simulink model "TDC_SMC_PD_S10x2810x29"  (R2025b)
settings: Solver=ode1be  StartTime=0.0  StopTime=1  FixedStep=0.001  MaxStep=0.01  RelTol=1e-3  EnableMultiTasking=on
values from neighbouring files (symbols this model uses):
  kd = 1.0245    [PD_final.m]
  kp = 16    [PD_final.m]
libraries: fod x3
settings Model: Creator=OMEN  LastModifiedBy=Wassim DJ
settings SolverCC: ZeroCrossControl=DisableAll  AlgebraicLoopSolver=TrustRegion
settings DataIOCC: ReturnWorkspaceOutputs=off
settings OptimizationCC: LifeSpan=inf
settings DebuggingCC: UnconnectedInputMsg=warning  UnconnectedOutputMsg=warning  UnconnectedLineMsg=warning  SFUnexpectedBacktrackingDiag=warning  SFNoUnconditionalDefaultTransitionDiag=warning  ArithmeticOperatorsInVariantConditions=warning
settings ModelReferenceCC: EnableRefExpFcnMdlSchedulingChecks=on
settings SFSimCC: SimUseLocalCustomCode=off  CustomCodeUndefinedFunction=UseInterfaceOnly
settings RTWCC: RTWUseLocalCustomCode=off  GPUComputeCapability=3.5  DLArmComputeVersion=19.05
settings CodeAppCC: StateflowObjectComments=on
settings GRTTargetCC: TargetLangStandard=C89/C90 (ANSI)
settings ConfigComp: CovMetricSettings=dw  CovSaveCumulativeToWorkspaceVar=on  CovSaveSingleToWorkspaceVar=on  CovExternalEMLEnable=off

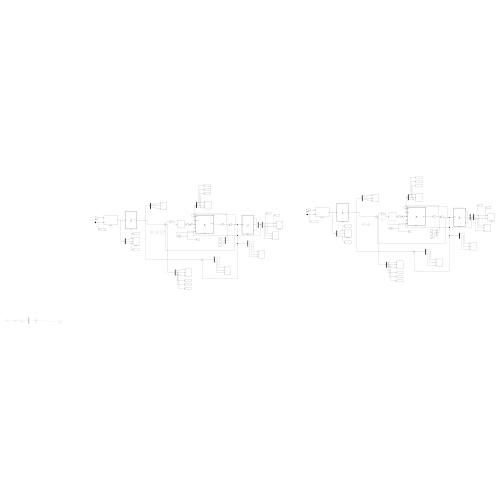
[thumbnail: Simulink's stored preview of the top-level diagram]
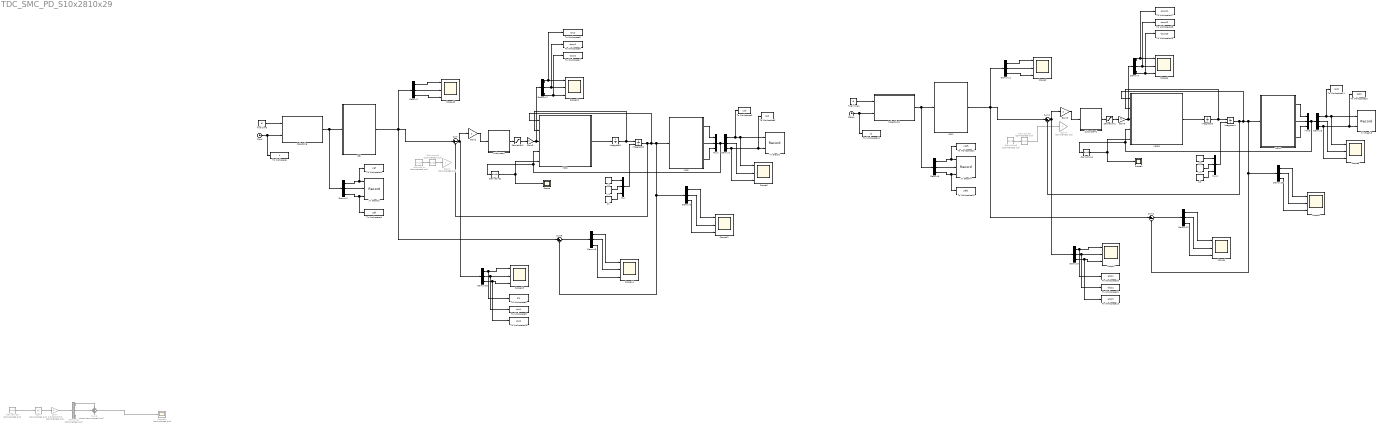
== system TDC_SMC_PD_S10x2810x29 ==
  Abs4 : Abs  Commented=on  SaturateOnIntegerOverflow=off
  Clock : Clock
  Clock1 : Clock
  Demux{1..12,17..18} (14 alike) : Demux  Outputs=3
  Demux22 : Demux  Commented=on  Outputs=3
  Derivative{,2..3,5..6} (5 alike) : Derivative  Commented=on
  Derivative1 : Derivative
  Derivative4 : Derivative
  Gain1 : Gain  Commented=on
  Gain2 : Gain
  Gain3 : Gain  Gain=3
  Gain4 : Gain  Commented=on
  Gain5 : Gain
  Gain6 : Gain  Gain=3
  Integrator1 : Integrator
  Integrator2 : Integrator  InitialConditionSource=external
  Integrator3 : Integrator
  Integrator4 : Integrator  InitialConditionSource=external
  Lam7 : Gain  Commented=on  Gain=0.000000005
  MDD : MATLAB Function  TreatAsAtomicUnit=on
  MDD1 : MATLAB Function  TreatAsAtomicUnit=on
  MGD : MATLAB Function  TreatAsAtomicUnit=on
  MGD1 : MATLAB Function  TreatAsAtomicUnit=on
  MGI : MATLAB Function  TreatAsAtomicUnit=on
  MGI1 : MATLAB Function  TreatAsAtomicUnit=on
  Mux{,1..3} (4 alike) : Mux  Inputs=3
  Saturation1 : Saturate  UpperLimit=15/12  LowerLimit=-15/12
  Saturation2 : Saturate  UpperLimit=15/12  LowerLimit=-15/12
  Scope : Scope
      settings: ActiveDisplayYMinimum=-0.16191  ActiveDisplayYMaximum=10.52394  DataLoggingVariableName=ScopeData4
  Scope1 : Scope
      settings: ActiveDisplayYMinimum=-0.16191  ActiveDisplayYMaximum=10.52394  DataLoggingVariableName=ScopeData2
  Scope{2..8,12..14,22..23} (12 alike) : Scope  NumInputPorts=3
      Scope12 settings: ActiveDisplayYMinimum=1.36342  ActiveDisplayYMaximum=5.69666
      Scope13 settings: ActiveDisplayYMinimum=-0.05003  ActiveDisplayYMaximum=2.21857  DataLoggingVariableName=ScopeData2
      Scope14 settings: ActiveDisplayYMinimum=-0.0016  ActiveDisplayYMaximum=0.00114  DataLoggingVariableName=ScopeData3
      Scope2 settings: ActiveDisplayYMinimum=1.36342  ActiveDisplayYMaximum=5.69666  DataLoggingVariableName=ScopeData3
      Scope22 settings: ActiveDisplayYMinimum=-3.78985  ActiveDisplayYMaximum=2.54114  DataLoggingVariableName=ScopeData3
      Scope23 settings: ActiveDisplayYMinimum=-0.02631  ActiveDisplayYMaximum=0.02531  DataLoggingVariableName=ScopeData4
      Scope3 settings: ActiveDisplayYMinimum=-0.05003  ActiveDisplayYMaximum=2.21857  DataLoggingVariableName=ScopeData4
      Scope4 settings: ActiveDisplayYMinimum=-0.0016  ActiveDisplayYMaximum=0.00114  DataLoggingVariableName=ScopeData5
      Scope5 settings: ActiveDisplayYMinimum=-0.31266  ActiveDisplayYMaximum=0.31251  DataLoggingVariableName=ScopeData4
      Scope6 settings: ActiveDisplayYMinimum=-4.18354  ActiveDisplayYMaximum=3.001  DataLoggingVariableName=ScopeData6
      Scope7 settings: ActiveDisplayYMinimum=-0.02631  ActiveDisplayYMaximum=0.02109  DataLoggingVariableName=ScopeData7
      Scope8 settings: ActiveDisplayYMinimum=-0.31266  ActiveDisplayYMaximum=0.31251  DataLoggingVariableName=ScopeData8
  Scope24 : Scope  Commented=on
      settings: ActiveDisplayYMinimum=-8E-7  ActiveDisplayYMaximum=7.5E-6
  Subsystem : Subsystem
  Subsystem1 : Subsystem
  Sum{,1..2,5} (4 alike) : Sum  Inputs=|+-
  Sum6 : Sum  Commented=on  Inputs=3
  To Workspace : ToWorkspace  VariableName=t  SampleTime=-1
      settings: Save2DSignal=2-D array (concatenate along first dimension)
  To Workspace1 : ToWorkspace  VariableName=xref  SampleTime=-1
      settings: Save2DSignal=2-D array (concatenate along first dimension)
  To Workspace10 : ToWorkspace  VariableName=alp2  SampleTime=-1
      settings: Save2DSignal=2-D array (concatenate along first dimension)
  To Workspace11 : ToWorkspace  VariableName=t1  SampleTime=-1
      settings: Save2DSignal=2-D array (concatenate along first dimension)
  To Workspace12 : ToWorkspace  VariableName=xref1  SampleTime=-1
      settings: Save2DSignal=2-D array (concatenate along first dimension)
  To Workspace13 : ToWorkspace  VariableName=alp13  SampleTime=-1
      settings: Save2DSignal=2-D array (concatenate along first dimension)
  To Workspace14 : ToWorkspace  VariableName=xpd1  SampleTime=-1
      settings: Save2DSignal=2-D array (concatenate along first dimension)
  To Workspace15 : ToWorkspace  VariableName=zpd1  SampleTime=-1
      settings: Save2DSignal=2-D array (concatenate along first dimension)
  To Workspace16 : ToWorkspace  VariableName=zref1  SampleTime=-1
      settings: Save2DSignal=2-D array (concatenate along first dimension)
  To Workspace17 : ToWorkspace  VariableName=coup11  SampleTime=-1
      settings: Save2DSignal=2-D array (concatenate along first dimension)
  To Workspace18 : ToWorkspace  VariableName=coup12  SampleTime=-1
      settings: Save2DSignal=2-D array (concatenate along first dimension)
  To Workspace19 : ToWorkspace  VariableName=coup13  SampleTime=-1
      settings: Save2DSignal=2-D array (concatenate along first dimension)
  To Workspace2 : ToWorkspace  VariableName=xpd  SampleTime=-1
      settings: Save2DSignal=2-D array (concatenate along first dimension)
  To Workspace20 : ToWorkspace  VariableName=alp11  SampleTime=-1
      settings: Save2DSignal=2-D array (concatenate along first dimension)
  To Workspace21 : ToWorkspace  VariableName=alp12  SampleTime=-1
      settings: Save2DSignal=2-D array (concatenate along first dimension)
  To Workspace3 : ToWorkspace  VariableName=zpd  SampleTime=-1
      settings: Save2DSignal=2-D array (concatenate along first dimension)
  To Workspace4 : ToWorkspace  VariableName=zref  SampleTime=-1
      settings: Save2DSignal=2-D array (concatenate along first dimension)
  To Workspace5 : ToWorkspace  VariableName=coup  SampleTime=-1
      settings: Save2DSignal=2-D array (concatenate along first dimension)
  To Workspace6 : ToWorkspace  VariableName=coup1  SampleTime=-1
      settings: Save2DSignal=2-D array (concatenate along first dimension)
  To Workspace7 : ToWorkspace  VariableName=coup2  SampleTime=-1
      settings: Save2DSignal=2-D array (concatenate along first dimension)
  To Workspace8 : ToWorkspace  VariableName=alp  SampleTime=-1
      settings: Save2DSignal=2-D array (concatenate along first dimension)
  To Workspace9 : ToWorkspace  VariableName=alp1  SampleTime=-1
      settings: Save2DSignal=2-D array (concatenate along first dimension)
  XY Graph1 : Record  NumPorts=2.0  FileSettingsInternal="{\"entries\":[{\"content\":{\"excelSettings\":{\"content\":{},\"type\":\"Streamout.ExcelSettings\"},\"parquetSettings\":{\"content\":{},\"type\":\"Streamout.ParquetSettings\"}},\"type\":\"Streamout.FileSettingStorage\",\"uuid\":\"\"}],\"packageUris\":[\"http:\\/\\/schema.mathworks.com\\/mf0\\/streamout_blocks\\/R2020a\"],\"version\":\"1.0\"}"  FrameSettings=[0, 0]  Layout=[1 1]  SignalsInternal="{\"entries\":[{\"content\":{\"signals\":[{\"content\":{\"blockPath\":[],\"dimensions\":[1],\"domain\":\"\",\"lineColor\":\"#a2142f\",\"plots\":[ 1 ],\"port\":1,\"signalID\":1,\"signalName\":\"Demux1:1\"},\"type\":\"RecordBlkView.Signal\",\"uuid\":\"\"},{\"content\":{\"blockPath\":[],\"dimensions\":[1],\"domain\":\"\",\"lineColor\":\"#139fff\",\"plots\":[ 1 ],\"port\":2,\"signalID\":2,\"signalName\":\"Demux1:3\"},\"type\":\"RecordBlkView.Signal\",\"uuid\":\"\"}]},\"type\":\"RecordBlkView.InputSignals\",\"uuid\":\"\"}],\"packageUris\":[\"http:\\/\\/schema.mathworks.com\\/mf0\\/streamout_blocks\\/R2020a\"],\"version\":\"1.0\"}"  VisualizationBindings="{\"xyplotplugin\":{\"info\":[{\"series\":[{\"bindingParametersList\":[{\"parameter\":\"X-Axis\",\"signalID\":1,\"signalName\":\"Demux1:1\"},{\"parameter\":\"Y-Axis\",\"signalID\":2,\"signalName\":\"Demux1:3\"}],\"seriesID\":0}],\"subplotID\":1}]}}"  CompatibilityTag=XY  st=-1
  XY Graph2 : Record  NumPorts=3.0  FileSettingsInternal="{\"entries\":[{\"content\":{\"excelSettings\":{\"content\":{},\"type\":\"Streamout.ExcelSettings\"},\"parquetSettings\":{\"content\":{},\"type\":\"Streamout.ParquetSettings\"}},\"type\":\"Streamout.FileSettingStorage\",\"uuid\":\"\"}],\"packageUris\":[\"http:\\/\\/schema.mathworks.com\\/mf0\\/streamout_blocks\\/R2020a\"],\"version\":\"1.0\"}"  FrameSettings=[0, 0, 0]  Layout=[1 1]  SignalsInternal="{\"entries\":[{\"content\":{\"signals\":[{\"content\":{\"blockPath\":[],\"dimensions\":[1,1],\"domain\":\"\",\"lineColor\":\"#a2142f\",\"plots\":[ 1 ],\"port\":1,\"signalID\":1,\"signalName\":\"Demux2:1\"},\"type\":\"RecordBlkView.Signal\",\"uuid\":\"\"},{\"content\":{\"blockPath\":[],\"dimensions\":[1,1],\"domain\":\"\",\"lineColor\":\"#139fff\",\"plots\":[ 1 ],\"port\":2,\"signalID\":2,\"signalName\":\"Demux2:2\"},\"type\":\"RecordBlkView.Signal\",\"uuid\":\"\"},{\"content\":{\"blockPath\":[],\"dimensions\":[1,1],\"domain\":\"\",\"lineColor\":\"#139fff\",\"lineWidth\":2,\"port\":3,\"signalID\":3,\"signalName\":\"Demux2:3\"},\"type\":\"RecordBlkView.Signal\",\"uuid\":\"\"}]},\"type\":\"RecordBlkView.InputSignals\",\"uuid\":\"\"}],\"packageUris\":[\"http:\\/\\/schema.mathworks.com\\/mf0\\/streamout_blocks\\/R2020a\"],\"version\":\"1.0\"}"  VisualizationBindings="{\"xyplotplugin\":{\"info\":[{\"series\":[{\"bindingParametersList\":[{\"parameter\":\"X-Axis\",\"signalID\":1,\"signalName\":\"Demux2:1\"},{\"parameter\":\"Y-Axis\",\"signalID\":2,\"signalName\":\"Demux2:2\"}],\"seriesID\":0}],\"subplotID\":1}]}}"  CompatibilityTag=XY  st=-1
  XY Graph3 : Record  NumPorts=2.0  FileSettingsInternal="{\"entries\":[{\"content\":{\"excelSettings\":{\"content\":{},\"type\":\"Streamout.ExcelSettings\"},\"parquetSettings\":{\"content\":{},\"type\":\"Streamout.ParquetSettings\"}},\"type\":\"Streamout.FileSettingStorage\",\"uuid\":\"\"}],\"packageUris\":[\"http:\\/\\/schema.mathworks.com\\/mf0\\/streamout_blocks\\/R2020a\"],\"version\":\"1.0\"}"  FrameSettings=[0, 0]  Layout=[1 1]  SignalsInternal="{\"entries\":[{\"content\":{\"signals\":[{\"content\":{\"blockPath\":[],\"dimensions\":[1],\"domain\":\"\",\"lineColor\":\"#a2142f\",\"plots\":[ 1 ],\"port\":1,\"signalID\":1,\"signalName\":\"Demux3:1\"},\"type\":\"RecordBlkView.Signal\",\"uuid\":\"\"},{\"content\":{\"blockPath\":[],\"dimensions\":[1],\"domain\":\"\",\"lineColor\":\"#139fff\",\"plots\":[ 1 ],\"port\":2,\"signalID\":2,\"signalName\":\"Demux3:3\"},\"type\":\"RecordBlkView.Signal\",\"uuid\":\"\"}]},\"type\":\"RecordBlkView.InputSignals\",\"uuid\":\"\"}],\"packageUris\":[\"http:\\/\\/schema.mathworks.com\\/mf0\\/streamout_blocks\\/R2020a\"],\"version\":\"1.0\"}"  VisualizationBindings="{\"xyplotplugin\":{\"info\":[{\"series\":[{\"bindingParametersList\":[{\"parameter\":\"X-Axis\",\"signalID\":1,\"signalName\":\"Demux3:1\"},{\"parameter\":\"Y-Axis\",\"signalID\":2,\"signalName\":\"Demux3:3\"}],\"seriesID\":0}],\"subplotID\":1}]}}"  CompatibilityTag=XY  st=-1
  XY Graph4 : Record  NumPorts=3.0  FileSettingsInternal="{\"entries\":[{\"content\":{\"excelSettings\":{\"content\":{},\"type\":\"Streamout.ExcelSettings\"},\"parquetSettings\":{\"content\":{},\"type\":\"Streamout.ParquetSettings\"}},\"type\":\"Streamout.FileSettingStorage\",\"uuid\":\"\"}],\"packageUris\":[\"http:\\/\\/schema.mathworks.com\\/mf0\\/streamout_blocks\\/R2020a\"],\"version\":\"1.0\"}"  FrameSettings=[0, 0, 0]  Layout=[1 1]  SignalsInternal="{\"entries\":[{\"content\":{\"signals\":[{\"content\":{\"blockPath\":[],\"dimensions\":[1,1],\"domain\":\"\",\"lineColor\":\"#a2142f\",\"plots\":[ 1 ],\"port\":1,\"signalID\":1,\"signalName\":\"Demux9:1\"},\"type\":\"RecordBlkView.Signal\",\"uuid\":\"\"},{\"content\":{\"blockPath\":[],\"dimensions\":[1,1],\"domain\":\"\",\"lineColor\":\"#139fff\",\"plots\":[ 1 ],\"port\":2,\"signalID\":2,\"signalName\":\"Demux9:2\"},\"type\":\"RecordBlkView.Signal\",\"uuid\":\"\"},{\"content\":{\"blockPath\":[],\"dimensions\":[1,1],\"domain\":\"\",\"lineColor\":\"#139fff\",\"lineWidth\":2,\"port\":3,\"signalID\":3,\"signalName\":\"Demux9:3\"},\"type\":\"RecordBlkView.Signal\",\"uuid\":\"\"}]},\"type\":\"RecordBlkView.InputSignals\",\"uuid\":\"\"}],\"packageUris\":[\"http:\\/\\/schema.mathworks.com\\/mf0\\/streamout_blocks\\/R2020a\"],\"version\":\"1.0\"}"  VisualizationBindings="{\"xyplotplugin\":{\"info\":[{\"series\":[{\"bindingParametersList\":[{\"parameter\":\"X-Axis\",\"signalID\":1,\"signalName\":\"Demux9:1\"},{\"parameter\":\"Y-Axis\",\"signalID\":2,\"signalName\":\"Demux9:2\"}],\"seriesID\":0}],\"subplotID\":1}]}}"  CompatibilityTag=XY  st=-1
  final time : Constant  Value=tf
  final time1 : Constant  Value=tf
  trajectoire : Subsystem
  trajectoire1 : Subsystem
  xi1 : Constant  Value=0.2821
  xi2 : Constant  Value=0.2821
  yi1 : Constant  Value=1.7584
  yi2 : Constant  Value=1.7584
  zi1 : Constant  Value=1.7584
  zi2 : Constant  Value=1.7584
  wires:
  Derivative1/1 -> MDD/5(dP), Scope/1
  Demux1/1 -> XY Graph1/1, Scope5/1, To Workspace2/1
  Demux1/3 -> Scope5/3, XY Graph1/2, To Workspace3/1
  Demux1/2 -> Scope5/2
  Integrator1/1 -> MDD/2(dalpha), Integrator2/1
  MDD/1(ddalpha) -> Integrator1/1
  xi1/1 -> Mux/1
  yi1/1 -> Mux/2
  zi1/1 -> Mux/3
  Mux/1 -> Integrator2/2
  MGI/1(alpha) -> Sum/1, Sum5/1, Demux7/1
  Sum/1 -> Gain2/1, Demux18/1
  Demux6/1 -> Scope12/1
  Demux6/3 -> Scope12/3
  Demux6/2 -> Scope12/2
  Integrator2/1 -> Sum/2, MDD/1(alpha), MGD/1(alpha), Demux6/1, Sum5/2
  Demux7/1 -> Scope13/1
  Demux7/3 -> Scope13/3
  Demux7/2 -> Scope13/2
  Demux8/1 -> Scope14/1
  Demux8/3 -> Scope14/3
  Demux8/2 -> Scope14/2
  Sum5/1 -> Demux8/1
  Mux1/1 -> MDD/4(P), Derivative1/1, Demux1/1
  MGD/1(X) -> Mux1/1
  Demux17/1 -> Scope22/1, To Workspace5/1
  Demux17/3 -> To Workspace7/1, Scope22/3
  Demux17/2 -> Scope22/2, To Workspace6/1
  Demux18/1 -> To Workspace8/1, Scope23/1
  Demux18/3 -> To Workspace10/1, Scope23/3
  Demux18/2 -> To Workspace9/1, Scope23/2
  final time/1 -> trajectoire/1(tf)
  Clock/1 -> To Workspace/1, trajectoire/2("time ")
  trajectoire/1(P) -> Demux2/1, MGI/1(P)
  MGD/2(Y) -> Mux1/2
  MGD/3(Z) -> Mux1/3
  Demux2/1 -> To Workspace1/1, XY Graph2/1
  Demux2/3 -> To Workspace4/1, XY Graph2/3
  Derivative/1 -> Derivative2/1
  Derivative2/1 -> Gain1/1
  Gain2/1 -> Subsystem/1(e)
  Saturation1/1 -> Gain3/1  "PD"
  Subsystem/1(T) -> Saturation1/1
  Gain3/1 -> Demux17/1, MDD/3(T)
  Demux2/2 -> XY Graph2/2
  Derivative5/1 -> Abs4/1
  Sum6/1 -> Scope24/1
  Abs4/1 -> Lam7/1
  Demux22/3 -> Sum6/3
  Lam7/1 -> Demux22/1
  Demux22/2 -> Sum6/2
  Demux22/1 -> Sum6/1
  Derivative3/1 -> Derivative6/1
  Saturation2/1 -> Gain6/1  "PD"
  Mux2/1 -> Integrator4/2
  Clock1/1 -> To Workspace11/1, trajectoire1/2("time ")
  MGD1/2(Y) -> Mux3/2
  Demux5/3 -> To Workspace13/1, Scope7/3
  Derivative4/1 -> MDD1/5(dP), Scope1/1
  MDD1/1(ddalpha) -> Integrator3/1
  Gain6/1 -> Demux4/1, MDD1/3(T)
  Demux9/1 -> To Workspace12/1, XY Graph4/1
  Gain5/1 -> Subsystem1/1(e)
  final time1/1 -> trajectoire1/1(tf)
  Demux12/2 -> Scope4/2
  MGD1/3(Z) -> Mux3/3
  Demux4/3 -> To Workspace19/1, Scope6/3
  Demux3/2 -> Scope8/2
  xi2/1 -> Mux2/1
  Demux11/1 -> Scope3/1
  Derivative6/1 -> Gain4/1
  Integrator4/1 -> Sum1/2, MDD1/1(alpha), MGD1/1(alpha), Demux10/1, Sum2/2
  Demux9/2 -> XY Graph4/2
  Demux11/2 -> Scope3/2
  Demux11/3 -> Scope3/3
  Demux12/1 -> Scope4/1
  Demux10/2 -> Scope2/2
  zi2/1 -> Mux2/3
  Demux3/3 -> Scope8/3, XY Graph3/2, To Workspace15/1
  Sum1/1 -> Gain5/1, Demux5/1
  Demux10/3 -> Scope2/3
  Demux10/1 -> Scope2/1
  Demux3/1 -> XY Graph3/1, Scope8/1, To Workspace14/1
  MGI1/1(alpha) -> Sum1/1, Sum2/1, Demux11/1
  Demux5/1 -> To Workspace20/1, Scope7/1
  trajectoire1/1(P) -> Demux9/1, MGI1/1(P)
  Demux5/2 -> To Workspace21/1, Scope7/2
  yi2/1 -> Mux2/2
  Subsystem1/1(T) -> Saturation2/1
  Demux4/2 -> Scope6/2, To Workspace18/1
  Mux3/1 -> MDD1/4(P), Derivative4/1, Demux3/1
  Integrator3/1 -> MDD1/2(dalpha), Integrator4/1
  Demux4/1 -> Scope6/1, To Workspace17/1
  MGD1/1(X) -> Mux3/1
  Demux12/3 -> Scope4/3
  Demux9/3 -> To Workspace16/1, XY Graph4/3
  Sum2/1 -> Demux12/1

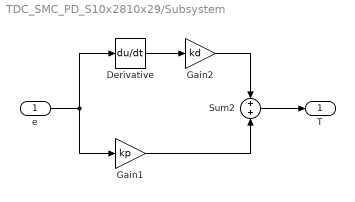
== system TDC_SMC_PD_S10x2810x29/Subsystem ==
  e : Inport
  Derivative : Derivative
  Gain1 : Gain  Gain=kp
  Gain2 : Gain  Gain=kd
  Sum2 : Sum
  T : Outport  VectorParamsAs1DForOutWhenUnconnected=off
  wires:
  e/1 -> Derivative/1, Gain1/1
  Derivative/1 -> Gain2/1
  Gain2/1 -> Sum2/1
  Gain1/1 -> Sum2/2
  Sum2/1 -> T/1

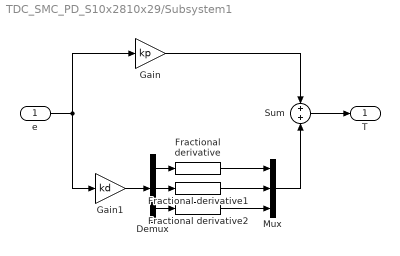
== system TDC_SMC_PD_S10x2810x29/Subsystem1 ==
  e : Inport
  Demux : Demux  Outputs=3
  Fractional derivative : fod/Fractional derivative  gam=mu  ww=[0.001; 1000]  n=5  nFod=off
      settings: SourceProductName=FOMCON Toolbox
  Fractional derivative1 : fod/Fractional derivative  gam=mu  ww=[0.001; 1000]  n=5  nFod=off
      settings: SourceProductName=FOMCON Toolbox
  Fractional derivative2 : fod/Fractional derivative  gam=mu  ww=[0.001; 1000]  n=5  nFod=off
      settings: SourceProductName=FOMCON Toolbox
  Gain : Gain  Gain=kp
  Gain1 : Gain  Gain=kd
  Mux : Mux  Inputs=3
  Sum : Sum
  T : Outport  VectorParamsAs1DForOutWhenUnconnected=off
  wires:
  Sum/1 -> T/1
  Gain/1 -> Sum/1
  e/1 -> Gain/1, Gain1/1
  Gain1/1 -> Demux/1
  Demux/1 -> Fractional derivative/1
  Demux/2 -> Fractional derivative1/1
  Demux/3 -> Fractional derivative2/1
  Fractional derivative1/1 -> Mux/2
  Fractional derivative/1 -> Mux/1
  Fractional derivative2/1 -> Mux/3
  Mux/1 -> Sum/2

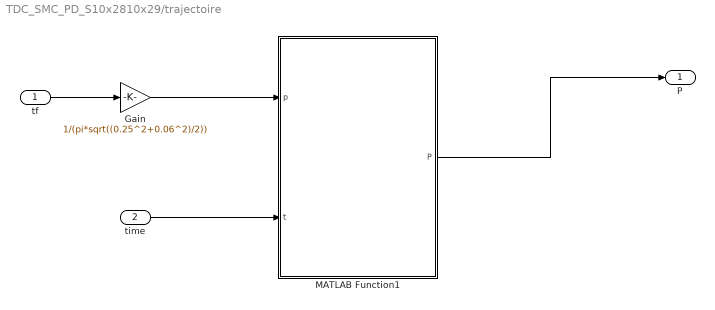
== system TDC_SMC_PD_S10x2810x29/trajectoire ==
  tf : Inport
  "time " : Inport  Port=2
  Gain : Gain  Gain=1/(pi*sqrt((0.25^2+0.06^2)/2))
  MATLAB Function1 : MATLAB Function  TreatAsAtomicUnit=on
  P : Outport  VectorParamsAs1DForOutWhenUnconnected=off
  wires:
  MATLAB Function1/1(P) -> P/1
  Gain/1 -> MATLAB Function1/1(p)
  "time "/1 -> MATLAB Function1/2(t)
  tf/1 -> Gain/1

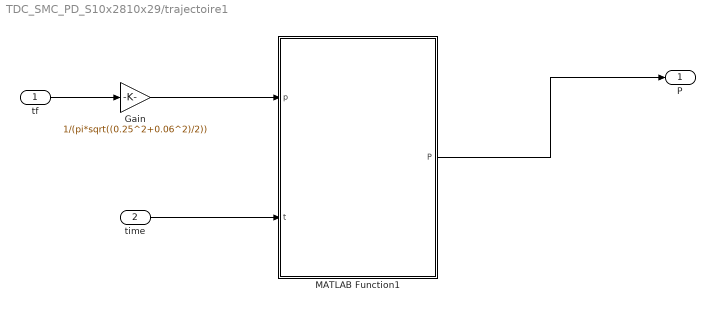
== system TDC_SMC_PD_S10x2810x29/trajectoire1 ==
  tf : Inport
  "time " : Inport  Port=2
  Gain : Gain  Gain=1/(pi*sqrt((0.25^2+0.06^2)/2))
  MATLAB Function1 : MATLAB Function  TreatAsAtomicUnit=on
  P : Outport  VectorParamsAs1DForOutWhenUnconnected=off
  wires:
  MATLAB Function1/1(P) -> P/1
  Gain/1 -> MATLAB Function1/1(p)
  "time "/1 -> MATLAB Function1/2(t)
  tf/1 -> Gain/1

== matlab function TDC_SMC_PD_S10x2810x29/MDD ==
  data: alpha input; ddalpha output; dalpha input; T input; P input; dP input
function ddalpha = MDD(alpha,dalpha,T,P,dP)
ddalpha = zeros(1,3);
phi = [0 2*pi/3 4*pi/3];
l1 = 0.205;
r = 0.15-0.024;
% these boudjedir table 2.1 page 30
mn = 0.042;
mfb = 0.028;
mb = 0.098;
mc = 0.015;
g = 9.81;
Im = 3.72e-5;
% documentation 0
% rotation matrix
R1 = [cos(phi(1)) -sin(phi(1)) 0;sin(phi(1)) cos(phi(1)) 0;0 0 1];
R2 = [cos(phi(2)) -sin(phi(2)) 0;sin(phi(2)) cos(phi(2)) 0;0 0 1]; 
R3 = [cos(phi(3)) -sin(phi(3)) 0;sin(phi(3)) cos(phi(3)) 0;0 0 1]; 

% eq 4.4
s1 = [P(1);P(2);P(3)]-R1*([r;0;0]+[l1*cos(alpha(1));0;l1*sin(alpha(1))]);    
s2 = [P(1);P(2);P(3)]-R2*([r;0;0]+[l1*cos(alpha(2));0;l1*sin(alpha(2))]); 
s3 = [P(1);P(2);P(3)]-R3*([r;0;0]+[l1*cos(alpha(3));0;l1*sin(alpha(3))]); 

% eq 4.9
b1 = R1*[-l1*sin(alpha(1));0;l1*cos(alpha(1))];
b2 = R2*[-l1*sin(alpha(2));0;l1*cos(alpha(2))];
b3 = R3*[-l1*sin(alpha(3));0;l1*cos(alpha(3))];

% eq 4.8
ds1 = [dP(1);dP(2);dP(3)]-R1*[-l1*sin(alpha(1));0;l1*cos(alpha(1))]*dalpha(1);
ds2 = [dP(1);dP(2);dP(3)]-R2*[-l1*sin(alpha(2));0;l1*cos(alpha(2))]*dalpha(2);
ds3 = [dP(1);dP(2);dP(3)]-R3*[-l1*sin(alpha(3));0;l1*cos(alpha(3))]*dalpha(3);

db1 = R1*[-l1*cos(alpha(1));0;-l1*sin(alpha(1))]*dalpha(1);
db2 = R2*[-l1*cos(alpha(2));0;-l1*sin(alpha(2))]*dalpha(2);
db3 = R3*[-l1*cos(alpha(3));0;-l1*sin(alpha(3))]*dalpha(3);

% eq 4.13
J = inv([s1';s2';s3'])*[s1'*b1 0 0;0 s2'*b2 0;0 0 s3'*b3];

dJ = inv([s1';s2';s3'])*(-[ds1';ds2';ds3']*J+[ds1'*b1+s1'*db1 0 0;0 ds2'*b2+s2'*db2 0;0 0 ds3'*b3+s3'*db3]);
% these boudjedir
% equa 2.42
mnt = mn+mfb;

% equa 2.49
Tgn = J'*mnt*[0 0 -g]';

% equa 2.44
mbr = mb+mc+2/3*mfb;

% equa 2.43
rgb = l1*(1/2*mb+mc+2/3*mfb)/mbr;

% equa 2.50
Tgb = rgb*mbr*g*[cos(alpha(1)) cos(alpha(2)) cos(alpha(3))]';

% equa 2.46
Ibc = l1^2*(mb/3+mc+2/3*mfb);
% equa 2.45
Ib = (Im*12^2+Ibc)*eye(3);

% equa 2.54
 ddalpha = (inv(Ib + mnt*J'*J)*(T - J'*mnt*dJ*dalpha' + Tgn + Tgb))';
if isnan(ddalpha)
    ddalpha = zeros(1,3);
end

== matlab function TDC_SMC_PD_S10x2810x29/trajectoire/MATLAB Function1 ==
  data: P output; p input; t input
function P   = trajectoire(p,t)


A=0.25;
B=0.06;
D=pi*sqrt((A^2+B^2)/2);



Xdes=0.25-A*(1-cos(pi*(t)/(p*D)));
Ydes=0*t;
Zdes=-0.43+B*sin(pi*(t)/(p*D));

dXdes=-A*pi/(p*D)*(sin(pi*(t)/(p*D)));
dYdes=0*t;
dZdes=B*pi/(p*D)*cos(pi*(t)/(p*D));

ddXdes=A*pi/(p*D)*pi/(p*D)*cos(pi*(t)/(p*D));
ddYdes=0*t;
ddZdes=-B*pi/(p*D)*pi/(p*D)*sin(pi*(t)/(p*D));

% Xdes=-0.25+A*(1-cos(pi*t/(p*D)));
% Ydes=0*t;
% Zdes=-0.43+B*sin(pi*t/(p*D));

P = [Xdes,Ydes,Zdes];
%dP = [dXdes,dYdes,dZdes];
%ddP = [ddXdes,ddYdes,ddZdes];

end

== matlab function TDC_SMC_PD_S10x2810x29/MDD1 ==
  data: alpha input; ddalpha output; dalpha input; T input; P input; dP input
function ddalpha = MDD(alpha,dalpha,T,P,dP)
ddalpha = zeros(1,3);
phi = [0 2*pi/3 4*pi/3];
l1 = 0.205;
r = 0.15-0.024;
% these boudjedir table 2.1 page 30
mn = 0.042;
mfb = 0.028;
mb = 0.098;
mc = 0.015;
g = 9.81;
Im = 3.72e-5;
% documentation 0
% rotation matrix
R1 = [cos(phi(1)) -sin(phi(1)) 0;sin(phi(1)) cos(phi(1)) 0;0 0 1];
R2 = [cos(phi(2)) -sin(phi(2)) 0;sin(phi(2)) cos(phi(2)) 0;0 0 1]; 
R3 = [cos(phi(3)) -sin(phi(3)) 0;sin(phi(3)) cos(phi(3)) 0;0 0 1]; 

% eq 4.4
s1 = [P(1);P(2);P(3)]-R1*([r;0;0]+[l1*cos(alpha(1));0;l1*sin(alpha(1))]);    
s2 = [P(1);P(2);P(3)]-R2*([r;0;0]+[l1*cos(alpha(2));0;l1*sin(alpha(2))]); 
s3 = [P(1);P(2);P(3)]-R3*([r;0;0]+[l1*cos(alpha(3));0;l1*sin(alpha(3))]); 

% eq 4.9
b1 = R1*[-l1*sin(alpha(1));0;l1*cos(alpha(1))];
b2 = R2*[-l1*sin(alpha(2));0;l1*cos(alpha(2))];
b3 = R3*[-l1*sin(alpha(3));0;l1*cos(alpha(3))];

% eq 4.8
ds1 = [dP(1);dP(2);dP(3)]-R1*[-l1*sin(alpha(1));0;l1*cos(alpha(1))]*dalpha(1);
ds2 = [dP(1);dP(2);dP(3)]-R2*[-l1*sin(alpha(2));0;l1*cos(alpha(2))]*dalpha(2);
ds3 = [dP(1);dP(2);dP(3)]-R3*[-l1*sin(alpha(3));0;l1*cos(alpha(3))]*dalpha(3);

db1 = R1*[-l1*cos(alpha(1));0;-l1*sin(alpha(1))]*dalpha(1);
db2 = R2*[-l1*cos(alpha(2));0;-l1*sin(alpha(2))]*dalpha(2);
db3 = R3*[-l1*cos(alpha(3));0;-l1*sin(alpha(3))]*dalpha(3);

% eq 4.13
J = inv([s1';s2';s3'])*[s1'*b1 0 0;0 s2'*b2 0;0 0 s3'*b3];

dJ = inv([s1';s2';s3'])*(-[ds1';ds2';ds3']*J+[ds1'*b1+s1'*db1 0 0;0 ds2'*b2+s2'*db2 0;0 0 ds3'*b3+s3'*db3]);
% these boudjedir
% equa 2.42
mnt = mn+mfb;

% equa 2.49
Tgn = J'*mnt*[0 0 -g]';

% equa 2.44
mbr = mb+mc+2/3*mfb;

% equa 2.43
rgb = l1*(1/2*mb+mc+2/3*mfb)/mbr;

% equa 2.50
Tgb = rgb*mbr*g*[cos(alpha(1)) cos(alpha(2)) cos(alpha(3))]';

% equa 2.46
Ibc = l1^2*(mb/3+mc+2/3*mfb);
% equa 2.45
Ib = (Im*12^2+Ibc)*eye(3);

% equa 2.54
 ddalpha = (inv(Ib + mnt*J'*J)*(T - J'*mnt*dJ*dalpha' + Tgn + Tgb))';
if isnan(ddalpha)
    ddalpha = zeros(1,3);
end

== matlab function TDC_SMC_PD_S10x2810x29/MGI ==
  data: P input; alpha output
function alpha = MGI(P)
phi = [0 2*pi/3 4*pi/3];
l1 = 0.205;
l2 = 0.380;
r = 0.15-0.024;
X = P(1,1);
Y = P(1,2);
Z = P(1,3);

A = zeros(1,3);
B = 2*Z*l1;
C = zeros(1,3);

for i=1:3
A(i) = 2*r*l1-2*X*l1*cos(phi(i))-2*Y*l1*sin(phi(i));
C(i) = l2^2-l1^2-r^2-X^2-Y^2-Z^2+2*X*r*cos(phi(i))+2*Y*r*sin(phi(i));    
end

alpha = zeros(1,3);
for i=1:3
    alpha(i) =  2*atan( (2*B+sqrt(abs(4*B^2+4*(A(i)+C(i))*(A(i)-C(i)))))/(2*(A(i)+C(i))));
    alpha(i) = double(alpha(i));
end

== matlab function TDC_SMC_PD_S10x2810x29/MGD1 ==
  data: alpha input; X output; Y output; Z output
function [X,Y,Z]  = MGD(alpha)

phi = [0 2*pi/3 4*pi/3];
l1 = 0.205;
l2 = 0.380;
r = 0.15-0.024;

D = zeros(1,3);
E = zeros(1,3);
F = zeros(1,3);
G = zeros(1,3);

for i=1:3
   D(i)=-l2^2+l1^2+r^2+2*r*l1*cos(alpha(i));
   E(i)=2*(r+l1*cos(alpha(i)))*cos(phi(i));
   F(i)=2*(r+l1*cos(alpha(i)))*sin(phi(i));
   G(i)=-2*l1*sin(alpha(i))  ;
end
% H1 = -(E(3)-E(1))*(G(2)-G(1))+(G(3)-G(1))*(E(2)-E(1));
% H2 = -(F(3)-F(1))*(E(2)-E(1))+(E(3)-E(1))*(F(2)-F(1));
% H3 = -(D(3)-D(1))*(E(2)-E(1))+(E(3)-E(1))*(D(2)-D(1));
% H4 = (D(3)-D(1))*(F(2)-F(1))-(F(3)-F(1))*(D(1)-D(2));
% H5 = -(G(3)-G(1))*(F(2)-F(1))-(F(3)-F(1))*(G(1)-G(2));

H1 = E(1)*G(2)-E(1)*G(3)-E(2)*G(1)+E(2)*G(3)+E(3)*G(1)-E(3)*G(2);
H2 = E(1)*(-F(2)+F(3))+E(2)*(F(1)-F(3))+E(3)*(-F(1)+F(2));
H3 = E(1)*(-D(2)+D(3))+E(2)*(D(1)-D(3))+E(3)*(-D(1)+D(2));
H4 = F(1)*(D(2)-D(3))+F(2)*(-D(1)+D(3))+F(3)*(D(1)-D(2));
H5 = F(1)*(-G(2)+G(3))+F(2)*(G(1)-G(3))+F(3)*(-G(1)+G(2));

L = ((H5^2+H1^2)/(H2^2))+1;
M = 2*(H5*H4+H1*H3)/(H2^2)-(H5*E(1)+H1*F(1))/H2-G(1);
N = (H4^2+H3^2)/H2^2-(H4*E(1)+H3*F(1))/H2+D(1);
Z = min((-M+sqrt(abs(M^2-4*L*N)))/(2*L),(-M-sqrt(abs(M^2-4*L*N)))/(2*L));
X = Z*(H5/H2)+(H4/H2);
Y = Z*(H1/H2)+(H3/H2);

X = double(X);
Y = double(Y);
Z = double(Z);

== matlab function TDC_SMC_PD_S10x2810x29/MGI1 ==
  data: P input; alpha output
function alpha = MGI(P)
phi = [0 2*pi/3 4*pi/3];
l1 = 0.205;
l2 = 0.380;
r = 0.15-0.024;
X = P(1,1);
Y = P(1,2);
Z = P(1,3);

A = zeros(1,3);
B = 2*Z*l1;
C = zeros(1,3);

for i=1:3
A(i) = 2*r*l1-2*X*l1*cos(phi(i))-2*Y*l1*sin(phi(i));
C(i) = l2^2-l1^2-r^2-X^2-Y^2-Z^2+2*X*r*cos(phi(i))+2*Y*r*sin(phi(i));    
end

alpha = zeros(1,3);
for i=1:3
    alpha(i) =  2*atan( (2*B+sqrt(abs(4*B^2+4*(A(i)+C(i))*(A(i)-C(i)))))/(2*(A(i)+C(i))));
    alpha(i) = double(alpha(i));
end

== matlab function TDC_SMC_PD_S10x2810x29/trajectoire1/MATLAB Function1 ==
  data: P output; p input; t input
function P   = trajectoire(p,t)


A=0.25;
B=0.06;
D=pi*sqrt((A^2+B^2)/2);



Xdes=0.25-A*(1-cos(pi*(t)/(p*D)));
Ydes=0*t;
Zdes=-0.43+B*sin(pi*(t)/(p*D));

dXdes=-A*pi/(p*D)*(sin(pi*(t)/(p*D)));
dYdes=0*t;
dZdes=B*pi/(p*D)*cos(pi*(t)/(p*D));

ddXdes=A*pi/(p*D)*pi/(p*D)*cos(pi*(t)/(p*D));
ddYdes=0*t;
ddZdes=-B*pi/(p*D)*pi/(p*D)*sin(pi*(t)/(p*D));

% Xdes=-0.25+A*(1-cos(pi*t/(p*D)));
% Ydes=0*t;
% Zdes=-0.43+B*sin(pi*t/(p*D));

P = [Xdes,Ydes,Zdes];
%dP = [dXdes,dYdes,dZdes];
%ddP = [ddXdes,ddYdes,ddZdes];

end

== matlab function TDC_SMC_PD_S10x2810x29/MGD ==
  data: alpha input; X output; Y output; Z output
function [X,Y,Z]  = MGD(alpha)

phi = [0 2*pi/3 4*pi/3];
l1 = 0.205;
l2 = 0.380;
r = 0.15-0.024;

D = zeros(1,3);
E = zeros(1,3);
F = zeros(1,3);
G = zeros(1,3);

for i=1:3
   D(i)=-l2^2+l1^2+r^2+2*r*l1*cos(alpha(i));
   E(i)=2*(r+l1*cos(alpha(i)))*cos(phi(i));
   F(i)=2*(r+l1*cos(alpha(i)))*sin(phi(i));
   G(i)=-2*l1*sin(alpha(i))  ;
end
% H1 = -(E(3)-E(1))*(G(2)-G(1))+(G(3)-G(1))*(E(2)-E(1));
% H2 = -(F(3)-F(1))*(E(2)-E(1))+(E(3)-E(1))*(F(2)-F(1));
% H3 = -(D(3)-D(1))*(E(2)-E(1))+(E(3)-E(1))*(D(2)-D(1));
% H4 = (D(3)-D(1))*(F(2)-F(1))-(F(3)-F(1))*(D(1)-D(2));
% H5 = -(G(3)-G(1))*(F(2)-F(1))-(F(3)-F(1))*(G(1)-G(2));

H1 = E(1)*G(2)-E(1)*G(3)-E(2)*G(1)+E(2)*G(3)+E(3)*G(1)-E(3)*G(2);
H2 = E(1)*(-F(2)+F(3))+E(2)*(F(1)-F(3))+E(3)*(-F(1)+F(2));
H3 = E(1)*(-D(2)+D(3))+E(2)*(D(1)-D(3))+E(3)*(-D(1)+D(2));
H4 = F(1)*(D(2)-D(3))+F(2)*(-D(1)+D(3))+F(3)*(D(1)-D(2));
H5 = F(1)*(-G(2)+G(3))+F(2)*(G(1)-G(3))+F(3)*(-G(1)+G(2));

L = ((H5^2+H1^2)/(H2^2))+1;
M = 2*(H5*H4+H1*H3)/(H2^2)-(H5*E(1)+H1*F(1))/H2-G(1);
N = (H4^2+H3^2)/H2^2-(H4*E(1)+H3*F(1))/H2+D(1);
Z = min((-M+sqrt(abs(M^2-4*L*N)))/(2*L),(-M-sqrt(abs(M^2-4*L*N)))/(2*L));
X = Z*(H5/H2)+(H4/H2);
Y = Z*(H1/H2)+(H3/H2);

X = double(X);
Y = double(Y);
Z = double(Z);
